simulink model "Q6"  (R2020b)
settings: Solver=VariableStepAuto  StartTime=0.0  StopTime=30  RelTol=1e-3
undefined symbols (not defined in the file): A_num, B_num, C_num, F, K_fast, L, P_inv, T_sol
settings Model: Creator=asus  LastModifiedBy=asus

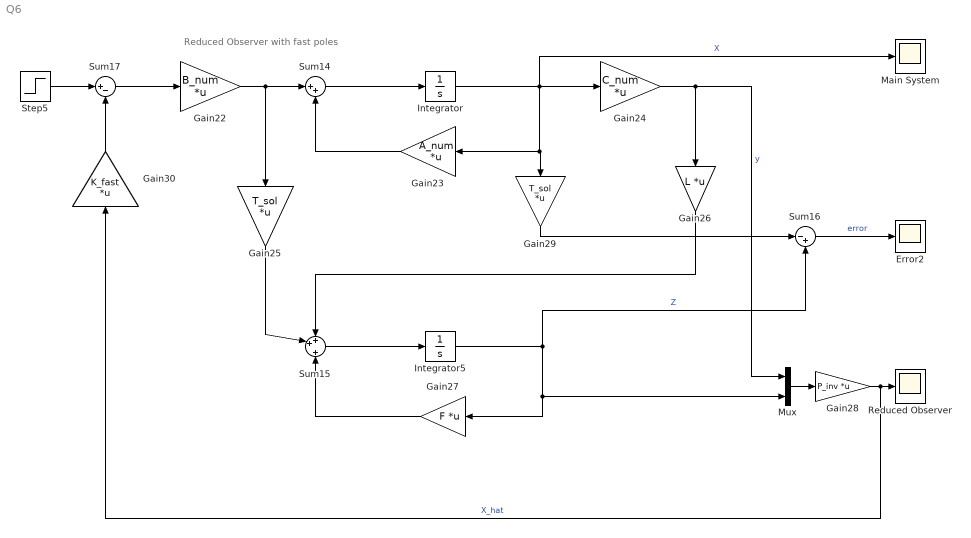
== system Q6 ==
  note: Reduced Observer with fast poles
  Error2 : Scope
  Gain22 : Gain  Gain=B_num  Multiplication=Matrix(K*u)
  Gain23 : Gain  Gain=A_num  Multiplication=Matrix(K*u)
  Gain24 : Gain  Gain=C_num  Multiplication=Matrix(K*u)
  Gain25 : Gain  Gain=T_sol  Multiplication=Matrix(K*u)
  Gain26 : Gain  Gain=L  Multiplication=Matrix(K*u)
  Gain27 : Gain  Gain=F  Multiplication=Matrix(K*u)
  Gain28 : Gain  Gain=P_inv  Multiplication=Matrix(K*u)
  Gain29 : Gain  Gain=T_sol  Multiplication=Matrix(K*u)
  Gain30 : Gain  Gain=K_fast  Multiplication=Matrix(K*u)
  Integrator : Integrator
  Integrator5 : Integrator
  Main System : Scope
  Mux : Mux  Inputs=2
  Reduced Observer : Scope
  Step5 : Step  SampleTime=0
  Sum14 : Sum  Inputs=|++
  Sum15 : Sum  Inputs=++|+
  Sum16 : Sum  Inputs=|-+
  Sum17 : Sum  Inputs=|+-
  wires:
  Integrator5/1 -> Sum16/2, Mux/2, Gain27/1  "Z"
  Gain22/1 -> Gain25/1, Sum14/1
  Mux/1 -> Gain28/1
  Sum16/1 -> Error2/1  "error"
  Gain28/1 -> Gain30/1, Reduced Observer/1  "X_hat"
  Step5/1 -> Sum17/1
  Gain27/1 -> Sum15/3
  Gain30/1 -> Sum17/2
  Gain25/1 -> Sum15/2
  Sum17/1 -> Gain22/1
  Sum14/1 -> Integrator/1
  Integrator/1 -> Gain29/1, Gain23/1, Gain24/1, Main System/1  "X"
  Gain29/1 -> Sum16/1
  Sum15/1 -> Integrator5/1
  Gain23/1 -> Sum14/2
  Gain24/1 -> Mux/1, Gain26/1  "y"
  Gain26/1 -> Sum15/1
